simulink model "powertrain"  (R2020b)
settings: Solver=FixedStepAuto  StartTime=0.0  StopTime=t(end)  RelTol=1e-3
PreLoadFcn:
  | C_sc = 1;
StartFcn:
  | C_sc = 1;
values from neighbouring files (symbols this model uses):
  D = 0    [model_fc.m]
  Ts = old_data.Ts    [model_fc.m]
undefined symbols (not defined in the file or in its folder): ANFIS, command, DiscIntNeverNeededParam, ECMS, Flight, in, Ion, Lithium, MPC, out, Tmpc, w
libraries: powerlib x25, neural x25, fuzblock x5, electricdrivelib x3, lib_converters x3, simulink x3, re_lib x1
(part 4 of 8)

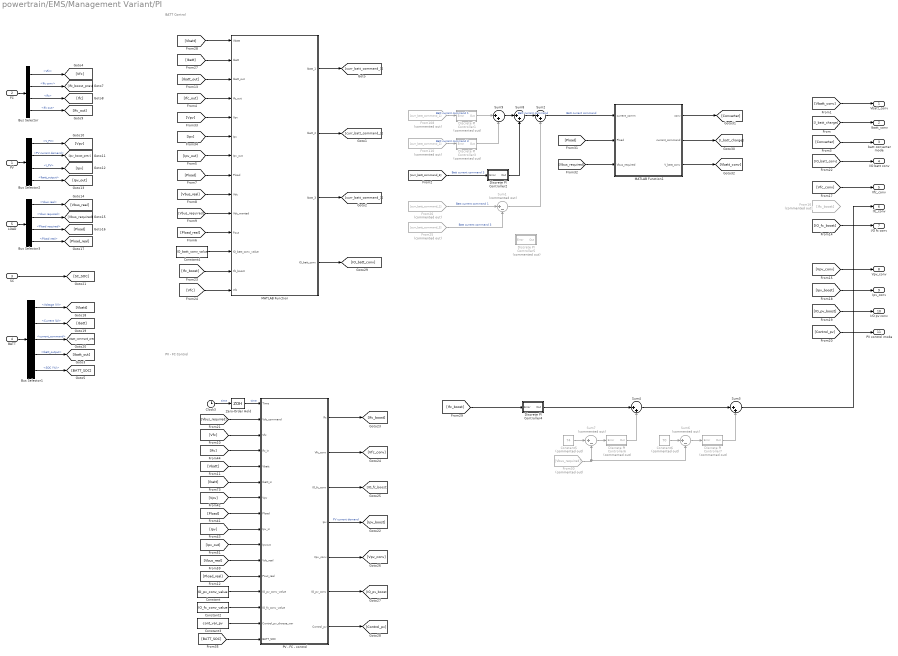
== system powertrain/EMS/Management Variant/PI ==
  note: PV - FC Control
  note: BATT Control
  PV : Inport
  FC : Inport  Port=2
  SC : Inport  Port=3
  BATT : Inport  Port=4
  LOAD : Inport  Port=5
  Bus Selector : BusSelector  OutputSignals=Vfc,Ifc conv,Ifc,Ifc out
  Bus Selector1 : BusSelector  OutputSignals=Voltage (V),Current (A),current_command,Ibatt_output,SOC (%)
  Bus Selector2 : BusSelector  OutputSignals=V_PV,PV current demand,I_PV,Ibatt_output
  Bus Selector3 : BusSelector  OutputSignals=Vbus real,Vbus required,Pload required,Pload real
  Clock3 : Clock
  Constant : Constant  Value=IO_pv_conv_value
  Constant2 : Constant  Value=IO_fc_conv_value
  Constant3 : Constant  Value=cont_var_pv
  Constant4 : Constant  Value=IO_batt_conv_value
  Constant5 : Constant  Commented=on  Value=74
  Constant6 : Constant  Commented=on  Value=70
  Discrete PI Controller1 : Subsystem  Commented=on  DialogController=POWERSYS.PowerSysDialog  mask(Discrete PI Controller){Kp=1, Ki=10, Par_Limits=[100 -100], Init=0, Ts=1e-4}
      mask prompts: Kp "Proportional gain (Kp):"; Ki "Integral gain (Ki):"; Par_Limits "Output limits: [ Upper   Lower ]"; Init "Output initial value:"; Ts "Sample time:"
      mask help: This block implements a discrete PI controller.
      mask init:
      | UpperLimit=Par_Limits(1);
      | LowerLimit=Par_Limits(2);
      | power_initmask();
      mask Help: This block is part of a subset of blocks in the Extras library that does not have documentation associated with it, other than the block mask description.
      mask Display: disp('PI');
  Discrete PI Controller2 : Subsystem  DialogController=POWERSYS.PowerSysDialog  mask(Discrete PI Controller){Kp=10, Ki=100, Par_Limits=[30 -4], Init=0, Ts=Ts}
      mask prompts: Kp "Proportional gain (Kp):"; Ki "Integral gain (Ki):"; Par_Limits "Output limits: [ Upper   Lower ]"; Init "Output initial value:"; Ts "Sample time:"
      mask help: This block implements a discrete PI controller.
      mask init:
      | UpperLimit=Par_Limits(1);
      | LowerLimit=Par_Limits(2);
      | power_initmask();
      mask Help: This block is part of a subset of blocks in the Extras library that does not have documentation associated with it, other than the block mask description.
      mask Display: disp('PI');
  Discrete PI Controller3 : Subsystem  Commented=on  DialogController=POWERSYS.PowerSysDialog  mask(Discrete PI Controller){Kp=10, Ki=1, Par_Limits=[100 -100], Init=0, Ts=1e-4}
      mask prompts: Kp "Proportional gain (Kp):"; Ki "Integral gain (Ki):"; Par_Limits "Output limits: [ Upper   Lower ]"; Init "Output initial value:"; Ts "Sample time:"
      mask help: This block implements a discrete PI controller.
      mask init:
      | UpperLimit=Par_Limits(1);
      | LowerLimit=Par_Limits(2);
      | power_initmask();
      mask Help: This block is part of a subset of blocks in the Extras library that does not have documentation associated with it, other than the block mask description.
      mask Display: disp('PI');
  Discrete PI Controller4 : Subsystem  DialogController=POWERSYS.PowerSysDialog  mask(Discrete PI Controller){Kp=10, Ki=10, Par_Limits=[33 0], Init=0, Ts=Ts}
      mask prompts: Kp "Proportional gain (Kp):"; Ki "Integral gain (Ki):"; Par_Limits "Output limits: [ Upper   Lower ]"; Init "Output initial value:"; Ts "Sample time:"
      mask help: This block implements a discrete PI controller.
      mask init:
      | UpperLimit=Par_Limits(1);
      | LowerLimit=Par_Limits(2);
      | power_initmask();
      mask Help: This block is part of a subset of blocks in the Extras library that does not have documentation associated with it, other than the block mask description.
      mask Display: disp('PI');
  Discrete PI Controller5 : Subsystem  Commented=on  DialogController=POWERSYS.PowerSysDialog  mask(Discrete PI Controller){Kp=10, Ki=10, Par_Limits=[50 -20], Init=0, Ts=1e-4}
      mask prompts: Kp "Proportional gain (Kp):"; Ki "Integral gain (Ki):"; Par_Limits "Output limits: [ Upper   Lower ]"; Init "Output initial value:"; Ts "Sample time:"
      mask help: This block implements a discrete PI controller.
      mask init:
      | UpperLimit=Par_Limits(1);
      | LowerLimit=Par_Limits(2);
      | power_initmask();
      mask Help: This block is part of a subset of blocks in the Extras library that does not have documentation associated with it, other than the block mask description.
      mask Display: disp('PI');
  Discrete PI Controller6 : Subsystem  Commented=on  DialogController=POWERSYS.PowerSysDialog  mask(Discrete PI Controller){Kp=10, Ki=10, Par_Limits=[40 0], Init=0, Ts=1e-4}
      mask prompts: Kp "Proportional gain (Kp):"; Ki "Integral gain (Ki):"; Par_Limits "Output limits: [ Upper   Lower ]"; Init "Output initial value:"; Ts "Sample time:"
      mask help: This block implements a discrete PI controller.
      mask init:
      | UpperLimit=Par_Limits(1);
      | LowerLimit=Par_Limits(2);
      | power_initmask();
      mask Help: This block is part of a subset of blocks in the Extras library that does not have documentation associated with it, other than the block mask description.
      mask Display: disp('PI');
  Discrete PI Controller7 : Subsystem  Commented=on  DialogController=POWERSYS.PowerSysDialog  mask(Discrete PI Controller){Kp=10, Ki=10, Par_Limits=[0 -40], Init=0, Ts=1e-4}
      mask prompts: Kp "Proportional gain (Kp):"; Ki "Integral gain (Ki):"; Par_Limits "Output limits: [ Upper   Lower ]"; Init "Output initial value:"; Ts "Sample time:"
      mask help: This block implements a discrete PI controller.
      mask init:
      | UpperLimit=Par_Limits(1);
      | LowerLimit=Par_Limits(2);
      | power_initmask();
      mask Help: This block is part of a subset of blocks in the Extras library that does not have documentation associated with it, other than the block mask description.
      mask Display: disp('PI');
  From108 : From  Commented=on  GotoTag=curr_batt_command_1
  From110 : From  Commented=on  GotoTag=curr_batt_command_2
  From16 : From  Commented=on  GotoTag=Ifc_boost
  From25 : From  Commented=on  GotoTag=curr_batt_command_3
  From26 : From  Commented=on  GotoTag=curr_batt_command_1
  From30 : From  Commented=on  GotoTag=Vbus_required
  MATLAB Function : MATLAB Function  TreatAsAtomicUnit=on
  MATLAB Function1 : MATLAB Function  TreatAsAtomicUnit=on
  PV - FC - control : MATLAB Function  TreatAsAtomicUnit=on
  Sum1 : Sum  Commented=on  Inputs=|+-
  Sum{2..4,8..9} (5 alike) : Sum  Inputs=|++
  Sum6 : Sum  Commented=on  Inputs=|+-
  Sum7 : Sum  Commented=on  Inputs=|+-
  Zero-Order Hold : ZeroOrderHold  SampleTime=Ts
  Vbatt_conv : Outport
  Ibatt_conv : Outport  Port=2
  batt converter mode : Outport  Port=3
  I/O batt conv : Outport  Port=4
  Vfc_conv : Outport  Port=5
  Ifc_conv : Outport  Port=6
  I/O fc conv : Outport  Port=7
  Vpv_conv : Outport  Port=8
  Ipv_conv : Outport  Port=9
  I/O pv conv : Outport  Port=10
  PV control mode : Outport  Port=11
  wires:
  [Ifc] -> PV - FC - control/4(Ifc_in)
  Bus Selector2/4 -> [Ipv_out]  "<Ibatt_output>"
  Bus Selector3/3 -> [Pload]  "<Pload required>"
  PV - FC - control/4(Ipv) -> [Ipv_boost]  "PV current demand"
  [Ipv_out] -> MATLAB Function/7(Ipv_out)
  [Control_pv] -> PV control mode/1
  From110/1 -> Discrete PI Controller3/1(Error)  "Batt current command 3"
  [IO_batt_conv] -> I/O batt conv/1
  Bus Selector/3 -> [Ifc]  "<Ifc>"
  [Vpv] -> PV - FC - control/7(Vpv)
  LOAD/1 -> Bus Selector3/1
  [Pload_real] -> PV - FC - control/12(Pout_real)
  Clock3/1 -> Zero-Order Hold/1  "time"
  [Vbus_required] -> MATLAB Function/10(Vdc_wanted)
  Constant5/1 -> Sum7/1
  Zero-Order Hold/1 -> PV - FC - control/1(Time)  "time"
  Sum8/1 -> Sum2/1  "Batt current command"
  [Pload] -> MATLAB Function/8(Pload)
  [Ipv] -> PV - FC - control/9(Ipv_in)
  [Vbus_real] -> PV - FC - control/11(Vdc_real)
  [Vbatt_conv] -> Vbatt_conv/1
  Constant3/1 -> PV - FC - control/15(Control_pv_choose_var)
  PV - FC - control/7(Control_pv) -> [Control_pv]
  MATLAB Function/4(IO_batt_conv) -> [IO_batt_conv]
  [Vbus_required] -> PV - FC - control/2(Vdc_command)
  Sum1/1 -> Sum2/2
  [Ipv_out] -> PV - FC - control/10(Ipvout)
  [Vfc_conv] -> Vfc_conv/1
  From25/1 -> Sum1/2  "Batt current command 3"
  [IO_pv_boost] -> I/O pv conv/1
  [Vfc] -> MATLAB Function/14(Vfc)
  [Ifc_boost] -> Discrete PI Controller4/1(Error)
  Bus Selector2/3 -> [Ipv]  "<I_PV>"
  [Ibatt] -> MATLAB Function/2(Ibatt)
  MATLAB Function/2(Ibatt_2) -> [curr_batt_command_2]
  MATLAB Function/1(Ibatt_1) -> [curr_batt_command_1]
  [Pload] -> MATLAB Function1/2(Pload)
  Bus Selector2/1 -> [Vpv]  "<V_PV>"
  Constant2/1 -> PV - FC - control/14(IO_fc_conv_value)
  Sum4/1 -> Sum3/1
  PV - FC - control/5(Vpv_conv) -> [Vpv_conv]
  MATLAB Function1/2(current_command) -> [I_batt_charge]
  Constant6/1 -> Sum6/1
  [Pload_real] -> MATLAB Function/11(Pout)
  Bus Selector1/1 -> [Vbatt]  "<Voltage (V)>"
  Sum2/1 -> MATLAB Function1/1(current_comm)  "Batt current command"
  [Vpv_conv] -> Vpv_conv/1
  [Ifc_boost] -> MATLAB Function/13(Ifc_boost)
  MATLAB Function1/3(V_batt_conv) -> [Vbatt_conv]
  Bus Selector1/2 -> [Ibatt]  "<Current (A)>"
  Bus Selector1/3 -> [Ibatt_command_pre]  "<current_command>"
  [Vbus_required] -> MATLAB Function1/3(Vbus_required)
  [Ifc_out] -> MATLAB Function/4(Ifc_out)
  [curr_batt_command_3] -> Discrete PI Controller2/1(Error)  "Batt current command 3"
  PV - FC - control/3(IO_fc_conv) -> [IO_fc_boost]
  PV/1 -> Bus Selector2/1
  From26/1 -> Sum1/1  "Batt current command 1"
  Sum6/1 -> Discrete PI Controller7/1(Error)
  [Vfc] -> PV - FC - control/3(Vfc)
  Bus Selector/4 -> [Ifc_out]  "<Ifc out>"
  PV - FC - control/2(Vfc_conv) -> [Vfc_conv]
  PV - FC - control/1(Ifc) -> [Ifc_boost]
  [I_batt_charge] -> Ibatt_conv/1
  FC/1 -> Bus Selector/1
  Bus Selector2/2 -> [Ipv_boost_prev]  "<PV current demand>"
  Bus Selector3/1 -> [Vbus_real]  "<Vbus real>"
  Bus Selector3/2 -> [Vbus_required]  "<Vbus required>"
  From30/1 -> Sum6/2, Sum7/2
  [Ipv_boost] -> Ipv_conv/1
  Sum7/1 -> Discrete PI Controller6/1(Error)
  Discrete PI Controller7/1(Out) -> Sum3/2
  [Vbatt] -> PV - FC - control/5(Vbatt)
  BATT/1 -> Bus Selector1/1
  PV - FC - control/6(IO_pv_conv) -> [IO_pv_boost]
  [Ibatt_out] -> MATLAB Function/3(Ibatt_out)
  SC/1 -> [SC_SOC]
  Bus Selector1/5 -> [BATT_SOC]  "<SOC (%)>"
  Bus Selector1/4 -> [Ibatt_out]  "<Ibatt_output>"
  [Vbatt] -> MATLAB Function/1(Vbatt)
  MATLAB Function1/1(conv) -> [Converter]
  Discrete PI Controller6/1(Out) -> Sum4/2
  Constant4/1 -> MATLAB Function/12(IO_batt_conv_value)
  [Ipv] -> MATLAB Function/6(Ipv)
  Bus Selector3/4 -> [Pload_real]  "<Pload real>"
  [IO_fc_boost] -> I/O fc conv/1
  Discrete PI Controller3/1(Out) -> Sum9/2
  MATLAB Function/3(Ibatt_3) -> [curr_batt_command_3]
  Sum3/1 -> Ifc_conv/1
  Discrete PI Controller2/1(Out) -> Sum8/2
  From108/1 -> Discrete PI Controller1/1(Error)  "Batt current command 1"
  [Pload] -> PV - FC - control/8(Pload)
  Bus Selector/2 -> [Ifc_boost_prev]  "<Ifc conv>"
  Discrete PI Controller1/1(Out) -> Sum9/1
  Constant/1 -> PV - FC - control/13(IO_pv_conv_value)
  Sum9/1 -> Sum8/1
  [Converter] -> batt converter mode/1
  [Vpv] -> MATLAB Function/5(Vpv)
  [Vbus_real] -> MATLAB Function/9(Vdc)
  [Ibatt] -> PV - FC - control/6(Ibatt_in)
  Bus Selector/1 -> [Vfc]  "<Vfc>"
  Discrete PI Controller4/1(Out) -> Sum4/1
  [BATT_SOC] -> PV - FC - control/16(BATT_SOC)

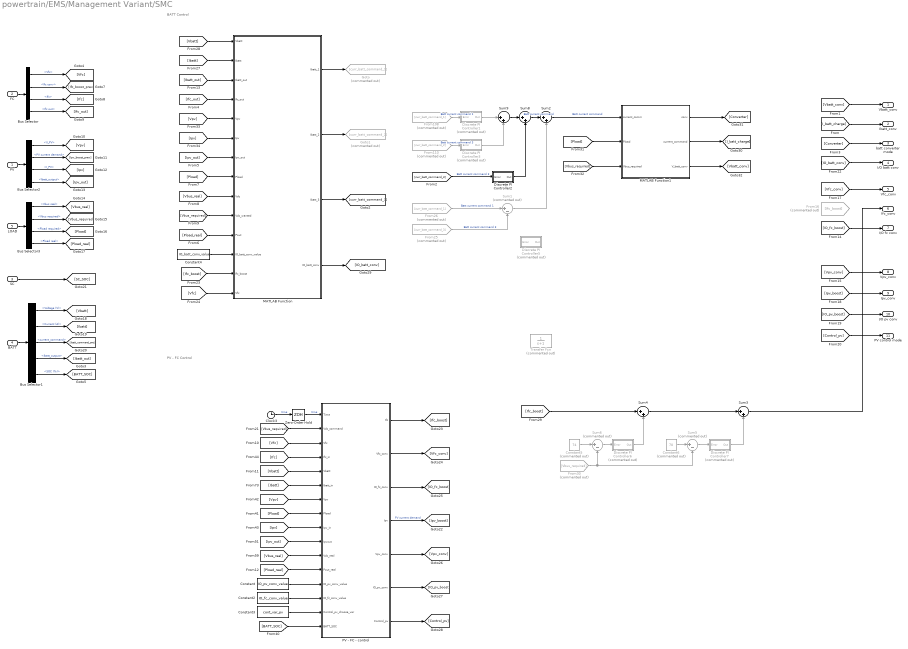
== system powertrain/EMS/Management Variant/SMC ==
  note: PV - FC Control
  note: BATT Control
  PV : Inport
  FC : Inport  Port=2
  SC : Inport  Port=3
  BATT : Inport  Port=4
  LOAD : Inport  Port=5
  Bus Selector : BusSelector  OutputSignals=Vfc,Ifc conv,Ifc,Ifc out
  Bus Selector1 : BusSelector  OutputSignals=Voltage (V),Current (A),current_command,Ibatt_output,SOC (%)
  Bus Selector2 : BusSelector  OutputSignals=V_PV,PV current demand,I_PV,Ibatt_output
  Bus Selector3 : BusSelector  OutputSignals=Vbus real,Vbus required,Pload required,Pload real
  Clock3 : Clock
  Constant : Constant  Value=IO_pv_conv_value
  Constant2 : Constant  Value=IO_fc_conv_value
  Constant3 : Constant  Value=cont_var_pv
  Constant4 : Constant  Value=IO_batt_conv_value
  Constant5 : Constant  Commented=on  Value=74
  Constant6 : Constant  Commented=on  Value=70
  Discrete PI Controller1 : Subsystem  Commented=on  DialogController=POWERSYS.PowerSysDialog  mask(Discrete PI Controller){Kp=1, Ki=10, Par_Limits=[100 -100], Init=0, Ts=1e-4}
      mask prompts: Kp "Proportional gain (Kp):"; Ki "Integral gain (Ki):"; Par_Limits "Output limits: [ Upper   Lower ]"; Init "Output initial value:"; Ts "Sample time:"
      mask help: This block implements a discrete PI controller.
      mask init:
      | UpperLimit=Par_Limits(1);
      | LowerLimit=Par_Limits(2);
      | power_initmask();
      mask Help: This block is part of a subset of blocks in the Extras library that does not have documentation associated with it, other than the block mask description.
      mask Display: disp('PI');
  Discrete PI Controller2 : Subsystem  DialogController=POWERSYS.PowerSysDialog  mask(Discrete PI Controller){Kp=10, Ki=100, Par_Limits=[30 -4], Init=0, Ts=Ts}
      mask prompts: Kp "Proportional gain (Kp):"; Ki "Integral gain (Ki):"; Par_Limits "Output limits: [ Upper   Lower ]"; Init "Output initial value:"; Ts "Sample time:"
      mask help: This block implements a discrete PI controller.
      mask init:
      | UpperLimit=Par_Limits(1);
      | LowerLimit=Par_Limits(2);
      | power_initmask();
      mask Help: This block is part of a subset of blocks in the Extras library that does not have documentation associated with it, other than the block mask description.
      mask Display: disp('PI');
  Discrete PI Controller3 : Subsystem  Commented=on  DialogController=POWERSYS.PowerSysDialog  mask(Discrete PI Controller){Kp=10, Ki=1, Par_Limits=[100 -100], Init=0, Ts=1e-4}
      mask prompts: Kp "Proportional gain (Kp):"; Ki "Integral gain (Ki):"; Par_Limits "Output limits: [ Upper   Lower ]"; Init "Output initial value:"; Ts "Sample time:"
      mask help: This block implements a discrete PI controller.
      mask init:
      | UpperLimit=Par_Limits(1);
      | LowerLimit=Par_Limits(2);
      | power_initmask();
      mask Help: This block is part of a subset of blocks in the Extras library that does not have documentation associated with it, other than the block mask description.
      mask Display: disp('PI');
  Discrete PI Controller5 : Subsystem  Commented=on  DialogController=POWERSYS.PowerSysDialog  mask(Discrete PI Controller){Kp=10, Ki=10, Par_Limits=[50 -20], Init=0, Ts=1e-4}
      mask prompts: Kp "Proportional gain (Kp):"; Ki "Integral gain (Ki):"; Par_Limits "Output limits: [ Upper   Lower ]"; Init "Output initial value:"; Ts "Sample time:"
      mask help: This block implements a discrete PI controller.
      mask init:
      | UpperLimit=Par_Limits(1);
      | LowerLimit=Par_Limits(2);
      | power_initmask();
      mask Help: This block is part of a subset of blocks in the Extras library that does not have documentation associated with it, other than the block mask description.
      mask Display: disp('PI');
  Discrete PI Controller6 : Subsystem  Commented=on  DialogController=POWERSYS.PowerSysDialog  mask(Discrete PI Controller){Kp=10, Ki=10, Par_Limits=[40 0], Init=0, Ts=Ts}
      mask prompts: Kp "Proportional gain (Kp):"; Ki "Integral gain (Ki):"; Par_Limits "Output limits: [ Upper   Lower ]"; Init "Output initial value:"; Ts "Sample time:"
      mask help: This block implements a discrete PI controller.
      mask init:
      | UpperLimit=Par_Limits(1);
      | LowerLimit=Par_Limits(2);
      | power_initmask();
      mask Help: This block is part of a subset of blocks in the Extras library that does not have documentation associated with it, other than the block mask description.
      mask Display: disp('PI');
  Discrete PI Controller7 : Subsystem  Commented=on  DialogController=POWERSYS.PowerSysDialog  mask(Discrete PI Controller){Kp=10, Ki=10, Par_Limits=[0 -40], Init=0, Ts=Ts}
      mask prompts: Kp "Proportional gain (Kp):"; Ki "Integral gain (Ki):"; Par_Limits "Output limits: [ Upper   Lower ]"; Init "Output initial value:"; Ts "Sample time:"
      mask help: This block implements a discrete PI controller.
      mask init:
      | UpperLimit=Par_Limits(1);
      | LowerLimit=Par_Limits(2);
      | power_initmask();
      mask Help: This block is part of a subset of blocks in the Extras library that does not have documentation associated with it, other than the block mask description.
      mask Display: disp('PI');
  From108 : From  Commented=on  GotoTag=curr_batt_command_1
  From110 : From  Commented=on  GotoTag=curr_batt_command_2
  From16 : From  Commented=on  GotoTag=Ifc_boost
  From25 : From  Commented=on  GotoTag=curr_batt_command_3
  From26 : From  Commented=on  GotoTag=curr_batt_command_1
  From30 : From  Commented=on  GotoTag=Vbus_required
  Goto : Goto  Commented=on  GotoTag=curr_batt_command_1
  Goto1 : Goto  Commented=on  GotoTag=curr_batt_command_2
  MATLAB Function : MATLAB Function  TreatAsAtomicUnit=on
  MATLAB Function1 : MATLAB Function  TreatAsAtomicUnit=on
  PV - FC - control : MATLAB Function  TreatAsAtomicUnit=on
  Sum1 : Sum  Commented=on  Inputs=|+-
  Sum{2..4,8..9} (5 alike) : Sum  Inputs=|++
  Sum5 : Sum  Commented=on  Inputs=|+-
  Sum6 : Sum  Commented=on  Inputs=|+-
  Transfer Fcn : TransferFcn  Commented=on  Denominator=[1 1]
  Zero-Order Hold : ZeroOrderHold  SampleTime=Ts
  Vbatt_conv : Outport
  Ibatt_conv : Outport  Port=2
  batt converter mode : Outport  Port=3
  I/O batt conv : Outport  Port=4
  Vfc_conv : Outport  Port=5
  Ifc_conv : Outport  Port=6
  I/O fc conv : Outport  Port=7
  Vpv_conv : Outport  Port=8
  Ipv_conv : Outport  Port=9
  I/O pv conv : Outport  Port=10
  PV control mode : Outport  Port=11
  wires:
  Sum2/1 -> MATLAB Function1/1(current_comm)  "Batt current command"
  Sum9/1 -> Sum8/1
  MATLAB Function/1(Ibatt_1) -> Goto/1
  MATLAB Function/2(Ibatt_2) -> Goto1/1
  MATLAB Function/3(Ibatt_3) -> [curr_batt_command_3]
  Discrete PI Controller1/1(Out) -> Sum9/1
  From108/1 -> Discrete PI Controller1/1(Error)  "Batt current command 1"
  Discrete PI Controller3/1(Out) -> Sum9/2
  [curr_batt_command_3] -> Discrete PI Controller2/1(Error)  "Batt current command 3"
  From110/1 -> Discrete PI Controller3/1(Error)  "Batt current command 3"
  [I_batt_charge] -> Ibatt_conv/1
  [Vbatt_conv] -> Vbatt_conv/1
  [Converter] -> batt converter mode/1
  SC/1 -> [SC_SOC]
  BATT/1 -> Bus Selector1/1
  FC/1 -> Bus Selector/1
  PV/1 -> Bus Selector2/1
  LOAD/1 -> Bus Selector3/1
  Bus Selector/1 -> [Vfc]  "<Vfc>"
  Bus Selector/3 -> [Ifc]  "<Ifc>"
  Bus Selector/4 -> [Ifc_out]  "<Ifc out>"
  Bus Selector2/1 -> [Vpv]  "<V_PV>"
  Bus Selector2/2 -> [Ipv_boost_prev]  "<PV current demand>"
  Bus Selector2/3 -> [Ipv]  "<I_PV>"
  Bus Selector2/4 -> [Ipv_out]  "<Ibatt_output>"
  Bus Selector3/1 -> [Vbus_real]  "<Vbus real>"
  Bus Selector3/2 -> [Vbus_required]  "<Vbus required>"
  Bus Selector3/3 -> [Pload]  "<Pload required>"
  Bus Selector3/4 -> [Pload_real]  "<Pload real>"
  Bus Selector/2 -> [Ifc_boost_prev]  "<Ifc conv>"
  [Vbus_required] -> MATLAB Function/10(Vdc_wanted)
  [Pload_real] -> MATLAB Function/11(Pout)
  [Vbus_real] -> MATLAB Function/9(Vdc)
  [Pload] -> MATLAB Function/8(Pload)
  [Ipv_out] -> MATLAB Function/7(Ipv_out)
  [Ifc_out] -> MATLAB Function/4(Ifc_out)
  [Vbatt] -> PV - FC - control/5(Vbatt)
  [BATT_SOC] -> PV - FC - control/16(BATT_SOC)
  Zero-Order Hold/1 -> PV - FC - control/1(Time)  "time"
  [Vpv] -> PV - FC - control/7(Vpv)
  PV - FC - control/4(Ipv) -> [Ipv_boost]  "PV current demand"
  [Ibatt] -> PV - FC - control/6(Ibatt_in)
  [Ipv] -> PV - FC - control/9(Ipv_in)
  [Pload] -> PV - FC - control/8(Pload)
  [Pload_real] -> PV - FC - control/12(Pout_real)
  Clock3/1 -> Zero-Order Hold/1  "time"
  [Vbus_required] -> PV - FC - control/2(Vdc_command)
  [Ipv_out] -> PV - FC - control/10(Ipvout)
  PV - FC - control/1(Ifc) -> [Ifc_boost]
  [Vfc] -> PV - FC - control/3(Vfc)
  [Vbus_real] -> PV - FC - control/11(Vdc_real)
  [Ifc] -> PV - FC - control/4(Ifc_in)
  [Vfc_conv] -> Vfc_conv/1
  [Vpv_conv] -> Vpv_conv/1
  PV - FC - control/2(Vfc_conv) -> [Vfc_conv]
  PV - FC - control/3(IO_fc_conv) -> [IO_fc_boost]
  PV - FC - control/5(Vpv_conv) -> [Vpv_conv]
  PV - FC - control/6(IO_pv_conv) -> [IO_pv_boost]
  Sum3/1 -> Ifc_conv/1
  [IO_fc_boost] -> I/O fc conv/1
  [Ipv_boost] -> Ipv_conv/1
  [IO_pv_boost] -> I/O pv conv/1
  PV - FC - control/7(Control_pv) -> [Control_pv]
  [Control_pv] -> PV control mode/1
  Constant/1 -> PV - FC - control/13(IO_pv_conv_value)
  Constant2/1 -> PV - FC - control/14(IO_fc_conv_value)
  Constant3/1 -> PV - FC - control/15(Control_pv_choose_var)
  [IO_batt_conv] -> I/O batt conv/1
  MATLAB Function/4(IO_batt_conv) -> [IO_batt_conv]
  Constant4/1 -> MATLAB Function/12(IO_batt_conv_value)
  [Ifc_boost] -> MATLAB Function/13(Ifc_boost)
  [Vfc] -> MATLAB Function/14(Vfc)
  From26/1 -> Sum1/1  "Batt current command 1"
  From25/1 -> Sum1/2  "Batt current command 3"
  [Ibatt] -> MATLAB Function/2(Ibatt)
  [Vbatt] -> MATLAB Function/1(Vbatt)
  Sum8/1 -> Sum2/1  "Batt current command"
  Sum1/1 -> Sum2/2
  Discrete PI Controller2/1(Out) -> Sum8/2
  Discrete PI Controller7/1(Out) -> Sum3/2
  Discrete PI Controller6/1(Out) -> Sum4/2
  [Ifc_boost] -> Sum4/1
  Sum4/1 -> Sum3/1
  Constant6/1 -> Sum5/1
  Sum5/1 -> Discrete PI Controller7/1(Error)
  Sum6/1 -> Discrete PI Controller6/1(Error)
  Constant5/1 -> Sum6/1
  From30/1 -> Sum5/2, Sum6/2
  MATLAB Function1/2(current_command) -> [I_batt_charge]
  MATLAB Function1/3(V_batt_conv) -> [Vbatt_conv]
  [Pload] -> MATLAB Function1/2(Pload)
  [Vbus_required] -> MATLAB Function1/3(Vbus_required)
  MATLAB Function1/1(conv) -> [Converter]
  Bus Selector1/1 -> [Vbatt]  "<Voltage (V)>"
  Bus Selector1/2 -> [Ibatt]  "<Current (A)>"
  Bus Selector1/3 -> [Ibatt_command_pre]  "<current_command>"
  Bus Selector1/4 -> [Ibatt_out]  "<Ibatt_output>"
  Bus Selector1/5 -> [BATT_SOC]  "<SOC (%)>"
  [Ibatt_out] -> MATLAB Function/3(Ibatt_out)
  [Vpv] -> MATLAB Function/5(Vpv)
  [Ipv] -> MATLAB Function/6(Ipv)

== system powertrain/EMS/Management Variant/ANFIS-ECMS/Discrete PI Controller1 ==
  note: Discrete PID Controller
  note: Pierre Giroux, Gilbert Sybille
      | Power System Simulation Laboratory
      | IREQ, Hydro-Quebc
  Error : Inport  SampleTime=Ts
  Discrete-Time Integrator : DiscreteIntegrator  InitialCondition=Init  SampleTime=Ts  LimitOutput=on  UpperSaturationLimit=UpperLimit  LowerSaturationLimit=LowerLimit  ICPrevOutput=DiscIntNeverNeededParam  ICPrevScaledInput=DiscIntNeverNeededParam
  Kp4 : Gain  Gain=Kp  SaturateOnIntegerOverflow=on  SampleTime=Ts  OutDataTypeStr=Inherit: Same as input  ParamDataTypeStr=Inherit: Same as input
  Kp5 : Gain  Gain=Ki  SaturateOnIntegerOverflow=on  SampleTime=Ts  OutDataTypeStr=Inherit: Same as input  ParamDataTypeStr=Inherit: Same as input
  Saturation2 : Saturate  UpperLimit=UpperLimit  LowerLimit=LowerLimit  SampleTime=Ts
  Sum6 : Sum  InputSameDT=on  SaturateOnIntegerOverflow=on  SampleTime=Ts  OutDataTypeStr=Inherit: Same as first input
  Zero-Order Hold : ZeroOrderHold  SampleTime=Ts
  Out : Outport  SampleTime=Ts  InitialOutput=0  VectorParamsAs1DForOutWhenUnconnected=off
  wires:
  Zero-Order Hold/1 -> Sum6/1
  Saturation2/1 -> Out/1
  Discrete-Time Integrator/1 -> Sum6/2
  Kp4/1 -> Zero-Order Hold/1
  Kp5/1 -> Discrete-Time Integrator/1
  Sum6/1 -> Saturation2/1
  Error/1 -> Kp5/1, Kp4/1

== system powertrain/EMS/Management Variant/ANFIS-ECMS/Discrete PI Controller2 ==
  note: Discrete PID Controller
  note: Pierre Giroux, Gilbert Sybille
      | Power System Simulation Laboratory
      | IREQ, Hydro-Quebc
  Error : Inport  SampleTime=Ts
  Discrete-Time Integrator : DiscreteIntegrator  InitialCondition=Init  SampleTime=Ts  LimitOutput=on  UpperSaturationLimit=UpperLimit  LowerSaturationLimit=LowerLimit  ICPrevOutput=DiscIntNeverNeededParam  ICPrevScaledInput=DiscIntNeverNeededParam
  Kp4 : Gain  Gain=Kp  SaturateOnIntegerOverflow=on  SampleTime=Ts  OutDataTypeStr=Inherit: Same as input  ParamDataTypeStr=Inherit: Same as input
  Kp5 : Gain  Gain=Ki  SaturateOnIntegerOverflow=on  SampleTime=Ts  OutDataTypeStr=Inherit: Same as input  ParamDataTypeStr=Inherit: Same as input
  Saturation2 : Saturate  UpperLimit=UpperLimit  LowerLimit=LowerLimit  SampleTime=Ts
  Sum6 : Sum  InputSameDT=on  SaturateOnIntegerOverflow=on  SampleTime=Ts  OutDataTypeStr=Inherit: Same as first input
  Zero-Order Hold : ZeroOrderHold  SampleTime=Ts
  Out : Outport  SampleTime=Ts  InitialOutput=0  VectorParamsAs1DForOutWhenUnconnected=off
  wires:
  Zero-Order Hold/1 -> Sum6/1
  Saturation2/1 -> Out/1
  Discrete-Time Integrator/1 -> Sum6/2
  Kp4/1 -> Zero-Order Hold/1
  Kp5/1 -> Discrete-Time Integrator/1
  Sum6/1 -> Saturation2/1
  Error/1 -> Kp5/1, Kp4/1

== system powertrain/EMS/Management Variant/ANFIS-ECMS/Discrete PI Controller3 ==
  note: Pierre Giroux, Gilbert Sybille
      | Power System Simulation Laboratory
      | IREQ, Hydro-Quebc
  note: Discrete PID Controller
  Error : Inport  SampleTime=Ts
  Discrete-Time Integrator : DiscreteIntegrator  InitialCondition=Init  SampleTime=Ts  LimitOutput=on  UpperSaturationLimit=UpperLimit  LowerSaturationLimit=LowerLimit  ICPrevOutput=DiscIntNeverNeededParam  ICPrevScaledInput=DiscIntNeverNeededParam
  Kp4 : Gain  Gain=Kp  SaturateOnIntegerOverflow=on  SampleTime=Ts  OutDataTypeStr=Inherit: Same as input  ParamDataTypeStr=Inherit: Same as input
  Kp5 : Gain  Gain=Ki  SaturateOnIntegerOverflow=on  SampleTime=Ts  OutDataTypeStr=Inherit: Same as input  ParamDataTypeStr=Inherit: Same as input
  Saturation2 : Saturate  UpperLimit=UpperLimit  LowerLimit=LowerLimit  SampleTime=Ts
  Sum6 : Sum  InputSameDT=on  SaturateOnIntegerOverflow=on  SampleTime=Ts  OutDataTypeStr=Inherit: Same as first input
  Zero-Order Hold : ZeroOrderHold  SampleTime=Ts
  Out : Outport  SampleTime=Ts  InitialOutput=0  VectorParamsAs1DForOutWhenUnconnected=off
  wires:
  Error/1 -> Kp4/1, Kp5/1
  Sum6/1 -> Saturation2/1
  Kp5/1 -> Discrete-Time Integrator/1
  Kp4/1 -> Zero-Order Hold/1
  Discrete-Time Integrator/1 -> Sum6/2
  Saturation2/1 -> Out/1
  Zero-Order Hold/1 -> Sum6/1

== system powertrain/EMS/Management Variant/ANFIS-ECMS/Time Delay Neural Network1 ==
  x : Inport  PortDimensions=1  SampleTime=0.01
      mask Display: e = 0.06;c1 = [120 230 180]/255;c2 = ([120 230 180]+0)/(256+128);c3 = ([120 230 180]+128)/(256+128);patch([0 1 1 0],[0 0 1 1],c1);patch([0 1 1 1-e 1-e 0+e],[0 0 1 1-e 0+e 0+e],c2);patch([0 0 1 1-e 0+e 0+e],[0 1 1 1-e 1-e 0+e],c3);plot([0 1 1 0 0],[0 0 1 1 0]);
  Layer 1 : Subsystem
      mask Display: e = 0.06;c1 = [120 150 230]/255;c2 = ([120 150 230]+0)/383;c3 = ([120 150 230]+128)/383;patch([0 1 1 0],[0 0 1 1],c1);patch([0 1 1 1-e 1-e 0+e],[0 0 1 1-e 0+e 0+e],c2);patch([0 0 1 1-e 0+e 0+e],[0 1 1 1-e 1-e 0+e],c3);plot([0 1 1 0 0],[0 0 1 1 0]);
  Layer 2 : Subsystem
      mask Display: e = 0.06;c1 = [120 150 230]/255;c2 = ([120 150 230]+0)/383;c3 = ([120 150 230]+128)/383;patch([0 1 1 0],[0 0 1 1],c1);patch([0 1 1 1-e 1-e 0+e],[0 0 1 1-e 0+e 0+e],c2);patch([0 0 1 1-e 0+e 0+e],[0 1 1 1-e 1-e 0+e],c3);plot([0 1 1 0 0],[0 0 1 1 0]);
  Process Input 1 : Subsystem
      mask Display: e = 0.06;c1 = [120 150 230]/255;c2 = ([120 150 230]+0)/383;c3 = ([120 150 230]+128)/383;patch([0 1 1 0],[0 0 1 1],c1);patch([0 1 1 1-e 1-e 0+e],[0 0 1 1-e 0+e 0+e],c2);patch([0 0 1 1-e 0+e 0+e],[0 1 1 1-e 1-e 0+e],c3);plot([0 1 1 0 0],[0 0 1 1 0]);
  Process Output 1 : Subsystem
      mask Display: e = 0.06;c1 = [120 150 230]/255;c2 = ([120 150 230]+0)/383;c3 = ([120 150 230]+128)/383;patch([0 1 1 0],[0 0 1 1],c1);patch([0 1 1 1-e 1-e 0+e],[0 0 1 1-e 0+e 0+e],c2);patch([0 0 1 1-e 0+e 0+e],[0 1 1 1-e 1-e 0+e],c3);plot([0 1 1 0 0],[0 0 1 1 0]);
  y : Outport  InitialOutput=0
      mask Display: e = 0.06;c1 = [120 230 180]/255;c2 = ([120 230 180]+0)/(256+128);c3 = ([120 230 180]+128)/(256+128);patch([0 1 1 0],[0 0 1 1],c1);patch([0 1 1 1-e 1-e 0+e],[0 0 1 1-e 0+e 0+e],c2);patch([0 0 1 1-e 0+e 0+e],[0 1 1 1-e 1-e 0+e],c3);plot([0 1 1 0 0],[0 0 1 1 0]);
  wires:
  Layer 2/1("a{2}") -> Process Output 1/1(a)
  [feedback1] -> Layer 2/1("a{1} ")
  Layer 1/1("a{1}") -> [feedback1]
  Process Input 1/1(p) -> Layer 1/1("p{1}")
  Process Output 1/1(y) -> y/1
  x/1 -> Process Input 1/1(x)

== system powertrain/EMS/Management Variant/Constant/Discrete PI Controller1 ==
  note: Pierre Giroux, Gilbert Sybille
      | Power System Simulation Laboratory
      | IREQ, Hydro-Quebc
  note: Discrete PID Controller
  Error : Inport  SampleTime=Ts
  Discrete-Time Integrator : DiscreteIntegrator  InitialCondition=Init  SampleTime=Ts  LimitOutput=on  UpperSaturationLimit=UpperLimit  LowerSaturationLimit=LowerLimit  ICPrevOutput=DiscIntNeverNeededParam  ICPrevScaledInput=DiscIntNeverNeededParam
  Kp4 : Gain  Gain=Kp  SaturateOnIntegerOverflow=on  SampleTime=Ts  OutDataTypeStr=Inherit: Same as input  ParamDataTypeStr=Inherit: Same as input
  Kp5 : Gain  Gain=Ki  SaturateOnIntegerOverflow=on  SampleTime=Ts  OutDataTypeStr=Inherit: Same as input  ParamDataTypeStr=Inherit: Same as input
  Saturation2 : Saturate  UpperLimit=UpperLimit  LowerLimit=LowerLimit  SampleTime=Ts
  Sum6 : Sum  InputSameDT=on  SaturateOnIntegerOverflow=on  SampleTime=Ts  OutDataTypeStr=Inherit: Same as first input
  Zero-Order Hold : ZeroOrderHold  SampleTime=Ts
  Out : Outport  SampleTime=Ts  InitialOutput=0  VectorParamsAs1DForOutWhenUnconnected=off
  wires:
  Error/1 -> Kp4/1, Kp5/1
  Sum6/1 -> Saturation2/1
  Kp5/1 -> Discrete-Time Integrator/1
  Kp4/1 -> Zero-Order Hold/1
  Discrete-Time Integrator/1 -> Sum6/2
  Saturation2/1 -> Out/1
  Zero-Order Hold/1 -> Sum6/1

== system powertrain/EMS/Management Variant/Constant/Discrete PI Controller2 ==
  note: Pierre Giroux, Gilbert Sybille
      | Power System Simulation Laboratory
      | IREQ, Hydro-Quebc
  note: Discrete PID Controller
  Error : Inport  SampleTime=Ts
  Discrete-Time Integrator : DiscreteIntegrator  InitialCondition=Init  SampleTime=Ts  LimitOutput=on  UpperSaturationLimit=UpperLimit  LowerSaturationLimit=LowerLimit  ICPrevOutput=DiscIntNeverNeededParam  ICPrevScaledInput=DiscIntNeverNeededParam
  Kp4 : Gain  Gain=Kp  SaturateOnIntegerOverflow=on  SampleTime=Ts  OutDataTypeStr=Inherit: Same as input  ParamDataTypeStr=Inherit: Same as input
  Kp5 : Gain  Gain=Ki  SaturateOnIntegerOverflow=on  SampleTime=Ts  OutDataTypeStr=Inherit: Same as input  ParamDataTypeStr=Inherit: Same as input
  Saturation2 : Saturate  UpperLimit=UpperLimit  LowerLimit=LowerLimit  SampleTime=Ts
  Sum6 : Sum  InputSameDT=on  SaturateOnIntegerOverflow=on  SampleTime=Ts  OutDataTypeStr=Inherit: Same as first input
  Zero-Order Hold : ZeroOrderHold  SampleTime=Ts
  Out : Outport  SampleTime=Ts  InitialOutput=0  VectorParamsAs1DForOutWhenUnconnected=off
  wires:
  Error/1 -> Kp4/1, Kp5/1
  Sum6/1 -> Saturation2/1
  Kp5/1 -> Discrete-Time Integrator/1
  Kp4/1 -> Zero-Order Hold/1
  Discrete-Time Integrator/1 -> Sum6/2
  Saturation2/1 -> Out/1
  Zero-Order Hold/1 -> Sum6/1

== system powertrain/EMS/Management Variant/Constant/Discrete PI Controller3 ==
  note: Discrete PID Controller
  note: Pierre Giroux, Gilbert Sybille
      | Power System Simulation Laboratory
      | IREQ, Hydro-Quebc
  Error : Inport  SampleTime=Ts
  Discrete-Time Integrator : DiscreteIntegrator  InitialCondition=Init  SampleTime=Ts  LimitOutput=on  UpperSaturationLimit=UpperLimit  LowerSaturationLimit=LowerLimit  ICPrevOutput=DiscIntNeverNeededParam  ICPrevScaledInput=DiscIntNeverNeededParam
  Kp4 : Gain  Gain=Kp  SaturateOnIntegerOverflow=on  SampleTime=Ts  OutDataTypeStr=Inherit: Same as input  ParamDataTypeStr=Inherit: Same as input
  Kp5 : Gain  Gain=Ki  SaturateOnIntegerOverflow=on  SampleTime=Ts  OutDataTypeStr=Inherit: Same as input  ParamDataTypeStr=Inherit: Same as input
  Saturation2 : Saturate  UpperLimit=UpperLimit  LowerLimit=LowerLimit  SampleTime=Ts
  Sum6 : Sum  InputSameDT=on  SaturateOnIntegerOverflow=on  SampleTime=Ts  OutDataTypeStr=Inherit: Same as first input
  Zero-Order Hold : ZeroOrderHold  SampleTime=Ts
  Out : Outport  SampleTime=Ts  InitialOutput=0  VectorParamsAs1DForOutWhenUnconnected=off
  wires:
  Zero-Order Hold/1 -> Sum6/1
  Saturation2/1 -> Out/1
  Discrete-Time Integrator/1 -> Sum6/2
  Kp4/1 -> Zero-Order Hold/1
  Kp5/1 -> Discrete-Time Integrator/1
  Sum6/1 -> Saturation2/1
  Error/1 -> Kp5/1, Kp4/1

== system powertrain/EMS/Management Variant/Constant/Discrete PI Controller5 ==
  note: Pierre Giroux, Gilbert Sybille
      | Power System Simulation Laboratory
      | IREQ, Hydro-Quebc
  note: Discrete PID Controller
  Error : Inport  SampleTime=Ts
  Discrete-Time Integrator : DiscreteIntegrator  InitialCondition=Init  SampleTime=Ts  LimitOutput=on  UpperSaturationLimit=UpperLimit  LowerSaturationLimit=LowerLimit  ICPrevOutput=DiscIntNeverNeededParam  ICPrevScaledInput=DiscIntNeverNeededParam
  Kp4 : Gain  Gain=Kp  SaturateOnIntegerOverflow=on  SampleTime=Ts  OutDataTypeStr=Inherit: Same as input  ParamDataTypeStr=Inherit: Same as input
  Kp5 : Gain  Gain=Ki  SaturateOnIntegerOverflow=on  SampleTime=Ts  OutDataTypeStr=Inherit: Same as input  ParamDataTypeStr=Inherit: Same as input
  Saturation2 : Saturate  UpperLimit=UpperLimit  LowerLimit=LowerLimit  SampleTime=Ts
  Sum6 : Sum  InputSameDT=on  SaturateOnIntegerOverflow=on  SampleTime=Ts  OutDataTypeStr=Inherit: Same as first input
  Zero-Order Hold : ZeroOrderHold  SampleTime=Ts
  Out : Outport  SampleTime=Ts  InitialOutput=0  VectorParamsAs1DForOutWhenUnconnected=off
  wires:
  Error/1 -> Kp4/1, Kp5/1
  Sum6/1 -> Saturation2/1
  Kp5/1 -> Discrete-Time Integrator/1
  Kp4/1 -> Zero-Order Hold/1
  Discrete-Time Integrator/1 -> Sum6/2
  Saturation2/1 -> Out/1
  Zero-Order Hold/1 -> Sum6/1

== system powertrain/EMS/Management Variant/Constant/Discrete PI Controller6 ==
  note: Discrete PID Controller
  note: Pierre Giroux, Gilbert Sybille
      | Power System Simulation Laboratory
      | IREQ, Hydro-Quebc
  Error : Inport  SampleTime=Ts
  Discrete-Time Integrator : DiscreteIntegrator  InitialCondition=Init  SampleTime=Ts  LimitOutput=on  UpperSaturationLimit=UpperLimit  LowerSaturationLimit=LowerLimit  ICPrevOutput=DiscIntNeverNeededParam  ICPrevScaledInput=DiscIntNeverNeededParam
  Kp4 : Gain  Gain=Kp  SaturateOnIntegerOverflow=on  SampleTime=Ts  OutDataTypeStr=Inherit: Same as input  ParamDataTypeStr=Inherit: Same as input
  Kp5 : Gain  Gain=Ki  SaturateOnIntegerOverflow=on  SampleTime=Ts  OutDataTypeStr=Inherit: Same as input  ParamDataTypeStr=Inherit: Same as input
  Saturation2 : Saturate  UpperLimit=UpperLimit  LowerLimit=LowerLimit  SampleTime=Ts
  Sum6 : Sum  InputSameDT=on  SaturateOnIntegerOverflow=on  SampleTime=Ts  OutDataTypeStr=Inherit: Same as first input
  Zero-Order Hold : ZeroOrderHold  SampleTime=Ts
  Out : Outport  SampleTime=Ts  InitialOutput=0  VectorParamsAs1DForOutWhenUnconnected=off
  wires:
  Zero-Order Hold/1 -> Sum6/1
  Saturation2/1 -> Out/1
  Discrete-Time Integrator/1 -> Sum6/2
  Kp4/1 -> Zero-Order Hold/1
  Kp5/1 -> Discrete-Time Integrator/1
  Sum6/1 -> Saturation2/1
  Error/1 -> Kp5/1, Kp4/1

== system powertrain/EMS/Management Variant/Constant/Discrete PI Controller7 ==
  note: Pierre Giroux, Gilbert Sybille
      | Power System Simulation Laboratory
      | IREQ, Hydro-Quebc
  note: Discrete PID Controller
  Error : Inport  SampleTime=Ts
  Discrete-Time Integrator : DiscreteIntegrator  InitialCondition=Init  SampleTime=Ts  LimitOutput=on  UpperSaturationLimit=UpperLimit  LowerSaturationLimit=LowerLimit  ICPrevOutput=DiscIntNeverNeededParam  ICPrevScaledInput=DiscIntNeverNeededParam
  Kp4 : Gain  Gain=Kp  SaturateOnIntegerOverflow=on  SampleTime=Ts  OutDataTypeStr=Inherit: Same as input  ParamDataTypeStr=Inherit: Same as input
  Kp5 : Gain  Gain=Ki  SaturateOnIntegerOverflow=on  SampleTime=Ts  OutDataTypeStr=Inherit: Same as input  ParamDataTypeStr=Inherit: Same as input
  Saturation2 : Saturate  UpperLimit=UpperLimit  LowerLimit=LowerLimit  SampleTime=Ts
  Sum6 : Sum  InputSameDT=on  SaturateOnIntegerOverflow=on  SampleTime=Ts  OutDataTypeStr=Inherit: Same as first input
  Zero-Order Hold : ZeroOrderHold  SampleTime=Ts
  Out : Outport  SampleTime=Ts  InitialOutput=0  VectorParamsAs1DForOutWhenUnconnected=off
  wires:
  Error/1 -> Kp4/1, Kp5/1
  Sum6/1 -> Saturation2/1
  Kp5/1 -> Discrete-Time Integrator/1
  Kp4/1 -> Zero-Order Hold/1
  Discrete-Time Integrator/1 -> Sum6/2
  Saturation2/1 -> Out/1
  Zero-Order Hold/1 -> Sum6/1

== system powertrain/EMS/Management Variant/D-ECMS/Discrete PI Controller1 ==
  note: Pierre Giroux, Gilbert Sybille
      | Power System Simulation Laboratory
      | IREQ, Hydro-Quebc
  note: Discrete PID Controller
  Error : Inport  SampleTime=Ts
  Discrete-Time Integrator : DiscreteIntegrator  InitialCondition=Init  SampleTime=Ts  LimitOutput=on  UpperSaturationLimit=UpperLimit  LowerSaturationLimit=LowerLimit  ICPrevOutput=DiscIntNeverNeededParam  ICPrevScaledInput=DiscIntNeverNeededParam
  Kp4 : Gain  Gain=Kp  SaturateOnIntegerOverflow=on  SampleTime=Ts  OutDataTypeStr=Inherit: Same as input  ParamDataTypeStr=Inherit: Same as input
  Kp5 : Gain  Gain=Ki  SaturateOnIntegerOverflow=on  SampleTime=Ts  OutDataTypeStr=Inherit: Same as input  ParamDataTypeStr=Inherit: Same as input
  Saturation2 : Saturate  UpperLimit=UpperLimit  LowerLimit=LowerLimit  SampleTime=Ts
  Sum6 : Sum  InputSameDT=on  SaturateOnIntegerOverflow=on  SampleTime=Ts  OutDataTypeStr=Inherit: Same as first input
  Zero-Order Hold : ZeroOrderHold  SampleTime=Ts
  Out : Outport  SampleTime=Ts  InitialOutput=0  VectorParamsAs1DForOutWhenUnconnected=off
  wires:
  Error/1 -> Kp4/1, Kp5/1
  Sum6/1 -> Saturation2/1
  Kp5/1 -> Discrete-Time Integrator/1
  Kp4/1 -> Zero-Order Hold/1
  Discrete-Time Integrator/1 -> Sum6/2
  Saturation2/1 -> Out/1
  Zero-Order Hold/1 -> Sum6/1

== system powertrain/EMS/Management Variant/D-ECMS/Discrete PI Controller2 ==
  note: Pierre Giroux, Gilbert Sybille
      | Power System Simulation Laboratory
      | IREQ, Hydro-Quebc
  note: Discrete PID Controller
  Error : Inport  SampleTime=Ts
  Discrete-Time Integrator : DiscreteIntegrator  InitialCondition=Init  SampleTime=Ts  LimitOutput=on  UpperSaturationLimit=UpperLimit  LowerSaturationLimit=LowerLimit  ICPrevOutput=DiscIntNeverNeededParam  ICPrevScaledInput=DiscIntNeverNeededParam
  Kp4 : Gain  Gain=Kp  SaturateOnIntegerOverflow=on  SampleTime=Ts  OutDataTypeStr=Inherit: Same as input  ParamDataTypeStr=Inherit: Same as input
  Kp5 : Gain  Gain=Ki  SaturateOnIntegerOverflow=on  SampleTime=Ts  OutDataTypeStr=Inherit: Same as input  ParamDataTypeStr=Inherit: Same as input
  Saturation2 : Saturate  UpperLimit=UpperLimit  LowerLimit=LowerLimit  SampleTime=Ts
  Sum6 : Sum  InputSameDT=on  SaturateOnIntegerOverflow=on  SampleTime=Ts  OutDataTypeStr=Inherit: Same as first input
  Zero-Order Hold : ZeroOrderHold  SampleTime=Ts
  Out : Outport  SampleTime=Ts  InitialOutput=0  VectorParamsAs1DForOutWhenUnconnected=off
  wires:
  Error/1 -> Kp4/1, Kp5/1
  Sum6/1 -> Saturation2/1
  Kp5/1 -> Discrete-Time Integrator/1
  Kp4/1 -> Zero-Order Hold/1
  Discrete-Time Integrator/1 -> Sum6/2
  Saturation2/1 -> Out/1
  Zero-Order Hold/1 -> Sum6/1

== system powertrain/EMS/Management Variant/D-ECMS/Discrete PI Controller3 ==
  note: Discrete PID Controller
  note: Pierre Giroux, Gilbert Sybille
      | Power System Simulation Laboratory
      | IREQ, Hydro-Quebc
  Error : Inport  SampleTime=Ts
  Discrete-Time Integrator : DiscreteIntegrator  InitialCondition=Init  SampleTime=Ts  LimitOutput=on  UpperSaturationLimit=UpperLimit  LowerSaturationLimit=LowerLimit  ICPrevOutput=DiscIntNeverNeededParam  ICPrevScaledInput=DiscIntNeverNeededParam
  Kp4 : Gain  Gain=Kp  SaturateOnIntegerOverflow=on  SampleTime=Ts  OutDataTypeStr=Inherit: Same as input  ParamDataTypeStr=Inherit: Same as input
  Kp5 : Gain  Gain=Ki  SaturateOnIntegerOverflow=on  SampleTime=Ts  OutDataTypeStr=Inherit: Same as input  ParamDataTypeStr=Inherit: Same as input
  Saturation2 : Saturate  UpperLimit=UpperLimit  LowerLimit=LowerLimit  SampleTime=Ts
  Sum6 : Sum  InputSameDT=on  SaturateOnIntegerOverflow=on  SampleTime=Ts  OutDataTypeStr=Inherit: Same as first input
  Zero-Order Hold : ZeroOrderHold  SampleTime=Ts
  Out : Outport  SampleTime=Ts  InitialOutput=0  VectorParamsAs1DForOutWhenUnconnected=off
  wires:
  Zero-Order Hold/1 -> Sum6/1
  Saturation2/1 -> Out/1
  Discrete-Time Integrator/1 -> Sum6/2
  Kp4/1 -> Zero-Order Hold/1
  Kp5/1 -> Discrete-Time Integrator/1
  Sum6/1 -> Saturation2/1
  Error/1 -> Kp5/1, Kp4/1

== system powertrain/EMS/Management Variant/D-ECMS/Discrete PI Controller5 ==
  note: Pierre Giroux, Gilbert Sybille
      | Power System Simulation Laboratory
      | IREQ, Hydro-Quebc
  note: Discrete PID Controller
  Error : Inport  SampleTime=Ts
  Discrete-Time Integrator : DiscreteIntegrator  InitialCondition=Init  SampleTime=Ts  LimitOutput=on  UpperSaturationLimit=UpperLimit  LowerSaturationLimit=LowerLimit  ICPrevOutput=DiscIntNeverNeededParam  ICPrevScaledInput=DiscIntNeverNeededParam
  Kp4 : Gain  Gain=Kp  SaturateOnIntegerOverflow=on  SampleTime=Ts  OutDataTypeStr=Inherit: Same as input  ParamDataTypeStr=Inherit: Same as input
  Kp5 : Gain  Gain=Ki  SaturateOnIntegerOverflow=on  SampleTime=Ts  OutDataTypeStr=Inherit: Same as input  ParamDataTypeStr=Inherit: Same as input
  Saturation2 : Saturate  UpperLimit=UpperLimit  LowerLimit=LowerLimit  SampleTime=Ts
  Sum6 : Sum  InputSameDT=on  SaturateOnIntegerOverflow=on  SampleTime=Ts  OutDataTypeStr=Inherit: Same as first input
  Zero-Order Hold : ZeroOrderHold  SampleTime=Ts
  Out : Outport  SampleTime=Ts  InitialOutput=0  VectorParamsAs1DForOutWhenUnconnected=off
  wires:
  Error/1 -> Kp4/1, Kp5/1
  Sum6/1 -> Saturation2/1
  Kp5/1 -> Discrete-Time Integrator/1
  Kp4/1 -> Zero-Order Hold/1
  Discrete-Time Integrator/1 -> Sum6/2
  Saturation2/1 -> Out/1
  Zero-Order Hold/1 -> Sum6/1

== system powertrain/EMS/Management Variant/D-ECMS/Discrete PI Controller6 ==
  note: Discrete PID Controller
  note: Pierre Giroux, Gilbert Sybille
      | Power System Simulation Laboratory
      | IREQ, Hydro-Quebc
  Error : Inport  SampleTime=Ts
  Discrete-Time Integrator : DiscreteIntegrator  InitialCondition=Init  SampleTime=Ts  LimitOutput=on  UpperSaturationLimit=UpperLimit  LowerSaturationLimit=LowerLimit  ICPrevOutput=DiscIntNeverNeededParam  ICPrevScaledInput=DiscIntNeverNeededParam
  Kp4 : Gain  Gain=Kp  SaturateOnIntegerOverflow=on  SampleTime=Ts  OutDataTypeStr=Inherit: Same as input  ParamDataTypeStr=Inherit: Same as input
  Kp5 : Gain  Gain=Ki  SaturateOnIntegerOverflow=on  SampleTime=Ts  OutDataTypeStr=Inherit: Same as input  ParamDataTypeStr=Inherit: Same as input
  Saturation2 : Saturate  UpperLimit=UpperLimit  LowerLimit=LowerLimit  SampleTime=Ts
  Sum6 : Sum  InputSameDT=on  SaturateOnIntegerOverflow=on  SampleTime=Ts  OutDataTypeStr=Inherit: Same as first input
  Zero-Order Hold : ZeroOrderHold  SampleTime=Ts
  Out : Outport  SampleTime=Ts  InitialOutput=0  VectorParamsAs1DForOutWhenUnconnected=off
  wires:
  Zero-Order Hold/1 -> Sum6/1
  Saturation2/1 -> Out/1
  Discrete-Time Integrator/1 -> Sum6/2
  Kp4/1 -> Zero-Order Hold/1
  Kp5/1 -> Discrete-Time Integrator/1
  Sum6/1 -> Saturation2/1
  Error/1 -> Kp5/1, Kp4/1

== system powertrain/EMS/Management Variant/D-ECMS/Discrete PI Controller7 ==
  note: Pierre Giroux, Gilbert Sybille
      | Power System Simulation Laboratory
      | IREQ, Hydro-Quebc
  note: Discrete PID Controller
  Error : Inport  SampleTime=Ts
  Discrete-Time Integrator : DiscreteIntegrator  InitialCondition=Init  SampleTime=Ts  LimitOutput=on  UpperSaturationLimit=UpperLimit  LowerSaturationLimit=LowerLimit  ICPrevOutput=DiscIntNeverNeededParam  ICPrevScaledInput=DiscIntNeverNeededParam
  Kp4 : Gain  Gain=Kp  SaturateOnIntegerOverflow=on  SampleTime=Ts  OutDataTypeStr=Inherit: Same as input  ParamDataTypeStr=Inherit: Same as input
  Kp5 : Gain  Gain=Ki  SaturateOnIntegerOverflow=on  SampleTime=Ts  OutDataTypeStr=Inherit: Same as input  ParamDataTypeStr=Inherit: Same as input
  Saturation2 : Saturate  UpperLimit=UpperLimit  LowerLimit=LowerLimit  SampleTime=Ts
  Sum6 : Sum  InputSameDT=on  SaturateOnIntegerOverflow=on  SampleTime=Ts  OutDataTypeStr=Inherit: Same as first input
  Zero-Order Hold : ZeroOrderHold  SampleTime=Ts
  Out : Outport  SampleTime=Ts  InitialOutput=0  VectorParamsAs1DForOutWhenUnconnected=off
  wires:
  Error/1 -> Kp4/1, Kp5/1
  Sum6/1 -> Saturation2/1
  Kp5/1 -> Discrete-Time Integrator/1
  Kp4/1 -> Zero-Order Hold/1
  Discrete-Time Integrator/1 -> Sum6/2
  Saturation2/1 -> Out/1
  Zero-Order Hold/1 -> Sum6/1

== system powertrain/EMS/Management Variant/ECAEMS/Discrete PI Controller1 ==
  note: Pierre Giroux, Gilbert Sybille
      | Power System Simulation Laboratory
      | IREQ, Hydro-Quebc
  note: Discrete PID Controller
  Error : Inport  SampleTime=Ts
  Discrete-Time Integrator : DiscreteIntegrator  InitialCondition=Init  SampleTime=Ts  LimitOutput=on  UpperSaturationLimit=UpperLimit  LowerSaturationLimit=LowerLimit  ICPrevOutput=DiscIntNeverNeededParam  ICPrevScaledInput=DiscIntNeverNeededParam
  Kp4 : Gain  Gain=Kp  SaturateOnIntegerOverflow=on  SampleTime=Ts  OutDataTypeStr=Inherit: Same as input  ParamDataTypeStr=Inherit: Same as input
  Kp5 : Gain  Gain=Ki  SaturateOnIntegerOverflow=on  SampleTime=Ts  OutDataTypeStr=Inherit: Same as input  ParamDataTypeStr=Inherit: Same as input
  Saturation2 : Saturate  UpperLimit=UpperLimit  LowerLimit=LowerLimit  SampleTime=Ts
  Sum6 : Sum  InputSameDT=on  SaturateOnIntegerOverflow=on  SampleTime=Ts  OutDataTypeStr=Inherit: Same as first input
  Zero-Order Hold : ZeroOrderHold  SampleTime=Ts
  Out : Outport  SampleTime=Ts  InitialOutput=0  VectorParamsAs1DForOutWhenUnconnected=off
  wires:
  Error/1 -> Kp4/1, Kp5/1
  Sum6/1 -> Saturation2/1
  Kp5/1 -> Discrete-Time Integrator/1
  Kp4/1 -> Zero-Order Hold/1
  Discrete-Time Integrator/1 -> Sum6/2
  Saturation2/1 -> Out/1
  Zero-Order Hold/1 -> Sum6/1

== system powertrain/EMS/Management Variant/ECAEMS/Discrete PI Controller2 ==
  note: Pierre Giroux, Gilbert Sybille
      | Power System Simulation Laboratory
      | IREQ, Hydro-Quebc
  note: Discrete PID Controller
  Error : Inport  SampleTime=Ts
  Discrete-Time Integrator : DiscreteIntegrator  InitialCondition=Init  SampleTime=Ts  LimitOutput=on  UpperSaturationLimit=UpperLimit  LowerSaturationLimit=LowerLimit  ICPrevOutput=DiscIntNeverNeededParam  ICPrevScaledInput=DiscIntNeverNeededParam
  Kp4 : Gain  Gain=Kp  SaturateOnIntegerOverflow=on  SampleTime=Ts  OutDataTypeStr=Inherit: Same as input  ParamDataTypeStr=Inherit: Same as input
  Kp5 : Gain  Gain=Ki  SaturateOnIntegerOverflow=on  SampleTime=Ts  OutDataTypeStr=Inherit: Same as input  ParamDataTypeStr=Inherit: Same as input
  Saturation2 : Saturate  UpperLimit=UpperLimit  LowerLimit=LowerLimit  SampleTime=Ts
  Sum6 : Sum  InputSameDT=on  SaturateOnIntegerOverflow=on  SampleTime=Ts  OutDataTypeStr=Inherit: Same as first input
  Zero-Order Hold : ZeroOrderHold  SampleTime=Ts
  Out : Outport  SampleTime=Ts  InitialOutput=0  VectorParamsAs1DForOutWhenUnconnected=off
  wires:
  Error/1 -> Kp4/1, Kp5/1
  Sum6/1 -> Saturation2/1
  Kp5/1 -> Discrete-Time Integrator/1
  Kp4/1 -> Zero-Order Hold/1
  Discrete-Time Integrator/1 -> Sum6/2
  Saturation2/1 -> Out/1
  Zero-Order Hold/1 -> Sum6/1

== system powertrain/EMS/Management Variant/ECAEMS/Discrete PI Controller3 ==
  note: Discrete PID Controller
  note: Pierre Giroux, Gilbert Sybille
      | Power System Simulation Laboratory
      | IREQ, Hydro-Quebc
  Error : Inport  SampleTime=Ts
  Discrete-Time Integrator : DiscreteIntegrator  InitialCondition=Init  SampleTime=Ts  LimitOutput=on  UpperSaturationLimit=UpperLimit  LowerSaturationLimit=LowerLimit  ICPrevOutput=DiscIntNeverNeededParam  ICPrevScaledInput=DiscIntNeverNeededParam
  Kp4 : Gain  Gain=Kp  SaturateOnIntegerOverflow=on  SampleTime=Ts  OutDataTypeStr=Inherit: Same as input  ParamDataTypeStr=Inherit: Same as input
  Kp5 : Gain  Gain=Ki  SaturateOnIntegerOverflow=on  SampleTime=Ts  OutDataTypeStr=Inherit: Same as input  ParamDataTypeStr=Inherit: Same as input
  Saturation2 : Saturate  UpperLimit=UpperLimit  LowerLimit=LowerLimit  SampleTime=Ts
  Sum6 : Sum  InputSameDT=on  SaturateOnIntegerOverflow=on  SampleTime=Ts  OutDataTypeStr=Inherit: Same as first input
  Zero-Order Hold : ZeroOrderHold  SampleTime=Ts
  Out : Outport  SampleTime=Ts  InitialOutput=0  VectorParamsAs1DForOutWhenUnconnected=off
  wires:
  Zero-Order Hold/1 -> Sum6/1
  Saturation2/1 -> Out/1
  Discrete-Time Integrator/1 -> Sum6/2
  Kp4/1 -> Zero-Order Hold/1
  Kp5/1 -> Discrete-Time Integrator/1
  Sum6/1 -> Saturation2/1
  Error/1 -> Kp5/1, Kp4/1
